simulink model "hitrostni_profili"  (Simulink 8.1)
settings: Solver=ode45  StartTime=0.0  StopTime=1800  MaxStep=1  RelTol=1e-3
values from neighbouring files (symbols this model uses):
  ETC_speed = [0.495937473176 0.496373873447 0.49680642819 0.497232592994 0.497650129408 0.498057004223 0.498451290329 0.498831082365 0.499194437912 0.499539351796 0.499863767467 0.500165625602 ... (17981 elements, 1x17981)]    [ETC_full.mat]
  ETC_time = [1.27562198744 1.37562198744 1.47562198744 1.57562198744 1.67562198744 1.77562198744 1.87562198744 1.97562198744 2.07562198744 2.17562198744 2.27562198744 2.37562198744 ... (17981 elements, 1x17981)]    [ETC_full.mat]
  WMTC_speed = [0.13809804916 0.140640874512 0.143161143435 0.145643612252 0.148074768295 0.150442285099 0.15273449872 0.154939979407 0.157047256677 0.159044735684 0.160920820235 0.162664234602 ... (17997 elements, 1x17997)]    [WMTC_full.mat]
  WMTC_time = [1.06312774212 1.16312774212 1.26312774212 1.36312774212 1.46312774212 1.56312774212 1.66312774212 1.76312774212 1.86312774212 1.96312774212 2.06312774212 2.16312774212 ... (17997 elements, 1x17997)]    [WMTC_full.mat]
libraries: simulink x12
settings Model: Creator=Mitja  LastModifiedBy=MitjaN
settings DebuggingCC: SaveWithParameterizedLinksMsg=none
settings HardwareCC: TargetHWDeviceType=32-bit Generic
settings GRTTargetCC: TargetFcnLib=ansi_tfl_tmw.mat

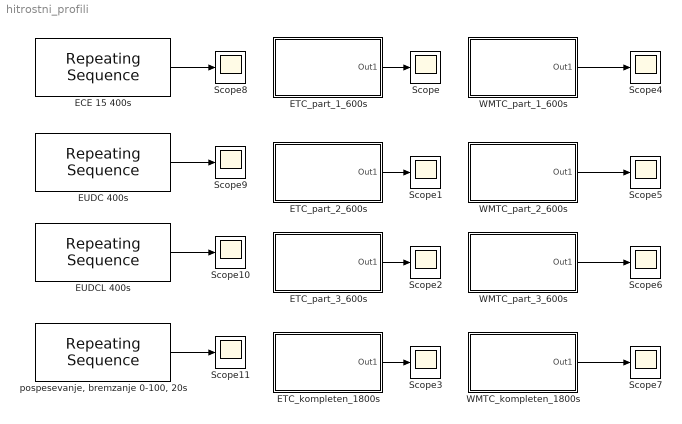
== system hitrostni_profili ==
  ECE 15 400s : simulink/Sources/Repeating Sequence  rep_seq_t=[0.0 11.3 15.0 23.2 28.2 48.9 60.8 85.2 95.9 117.2 142.8 154.8 162.9 176.0 188.0 200.0]  rep_seq_y=[0.0 0.0 5.0 5.0 0.0 0.0 32.0 32.0 0.0 0.0 50.0 50.0 35.0 35.0 0.0 0.0]
  ETC_kompleten_1800s : Subsystem  InitFcn=load('ETC_full.mat')
  ETC_part_1_600s : Subsystem  InitFcn=load('ETC_part_1.mat')
  ETC_part_2_600s : Subsystem  InitFcn=load('ETC_part_2.mat')
  ETC_part_3_600s : Subsystem  InitFcn=load('ETC_part_3.mat')
  EUDC 400s : simulink/Sources/Repeating Sequence  rep_seq_t=[0.0 20.5128 24.359 30.7692 34.6154 43.5897 60.2564 111.538 115.385 119.231 188.462 193.59 194.872 200.0 250.0 284.615 315.385 334.615 346.154 364.103 371.795 379.487 400.0]  rep_seq_y=[0.0 0.0 7.0 19.0 26.0 42.0 70.0 70.0 58.2775 50.0 50.0 58.2775 60.9569 70.0 70.0 100.0 100.0 120.0 120.0 71.0048 37.512 0.0 0.0]
  EUDCL 400s : simulink/Sources/Repeating Sequence  rep_seq_t=|  rep_seq_y=|
      rep_seq_t=|
      | [    0.00000000000000e+000
      |     20.5128000000000e+000
      |     23.0769000000000e+000
      |     28.2051000000000e+000
      |     35.8974000000000e+000
      |     46.1538000000000e+000
      |     61.5385000000000e+000
      |     111.538000000000e+000
      |     115.385000000000e+000
      |     119.231000000000e+000
      |     188.462000000000e+000
      |     193.590000000000e+000
      |     201.282000000000e+000
      |     251.282000000000e+000
      |     274.359000000000e+000
      |     357.692000000000e+000
      |     365.385000000000e+000
      |     379.487000000000e+000
      |     400.000000000000e+000]
      rep_seq_y=|
      | [    0.00000000000000e+000
      |     0.00000000000000e+000
      |     11.0048000000000e+000
      |     18.6603000000000e+000
      |     34.9282000000000e+000
      |     49.7608000000000e+000
      |     70.0000000000000e+000
      |     70.0000000000000e+000
      |     59.3301000000000e+000
      |     50.0000000000000e+000
      |     50.0000000000000e+000
      |     60.2871000000000e+000
      |     70.0000000000000e+000
      |     70.0000000000000e+000
      |     90.0000000000000e+000
      |     90.0000000000000e+000
      |     67.4641000000000e+000
      |     0.00000000000000e+000
      |     0.00000000000000e+000]
  Scope{,1..11} (12 alike) : Scope
      Scope10 settings: SaveName=ScopeData10
      Scope11 settings: SaveName=ScopeData11
      Scope2 settings: SaveName=ScopeData2
      Scope3 settings: SaveName=ScopeData3
      Scope4 settings: SaveName=ScopeData4
      Scope5 settings: SaveName=ScopeData5
      Scope6 settings: SaveName=ScopeData6
      Scope7 settings: SaveName=ScopeData7
      Scope8 settings: SaveName=ScopeData8
      Scope9 settings: SaveName=ScopeData9
  WMTC_kompleten_1800s : Subsystem  InitFcn=load('WMTC_full.mat')
  WMTC_part_1_600s : Subsystem  InitFcn=load('WMTC_part_1.mat')
  WMTC_part_2_600s : Subsystem  InitFcn=load('WMTC_part_2.mat')
  WMTC_part_3_600s : Subsystem  InitFcn=load('WMTC_part_3.mat')
  "pospesevanje, bremzanje 0-100, 20s" : simulink/Sources/Repeating Sequence  rep_seq_t=[0 1 11 15 17 20]  rep_seq_y=[0 0 100 100 0 0]
  wires:
  ETC_part_1_600s/1(Out1) -> Scope/1
  WMTC_kompleten_1800s/1(Out1) -> Scope7/1
  WMTC_part_3_600s/1(Out1) -> Scope6/1
  WMTC_part_2_600s/1(Out1) -> Scope5/1
  WMTC_part_1_600s/1(Out1) -> Scope4/1
  ETC_part_2_600s/1(Out1) -> Scope1/1
  ETC_part_3_600s/1(Out1) -> Scope2/1
  ETC_kompleten_1800s/1(Out1) -> Scope3/1
  ECE 15 400s/1 -> Scope8/1
  EUDC 400s/1 -> Scope9/1
  EUDCL 400s/1 -> Scope10/1
  "pospesevanje, bremzanje 0-100, 20s"/1 -> Scope11/1

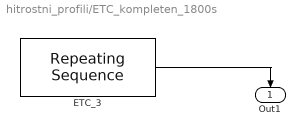
== system hitrostni_profili/ETC_kompleten_1800s ==
  ETC_3 : simulink/Sources/Repeating Sequence  rep_seq_t=[ETC_time]  rep_seq_y=[ETC_speed]
  Out1 : Outport
  wires:
  ETC_3/1 -> Out1/1

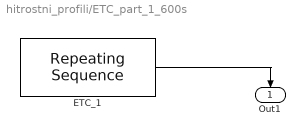
== system hitrostni_profili/ETC_part_1_600s ==
  ETC_1 : simulink/Sources/Repeating Sequence  rep_seq_t=ETC_1_time  rep_seq_y=ETC_1_speed
  Out1 : Outport
  wires:
  ETC_1/1 -> Out1/1

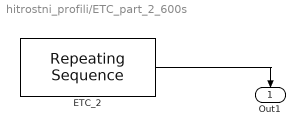
== system hitrostni_profili/ETC_part_2_600s ==
  ETC_2 : simulink/Sources/Repeating Sequence  rep_seq_t=ETC_2_time  rep_seq_y=ETC_2_speed
  Out1 : Outport
  wires:
  ETC_2/1 -> Out1/1

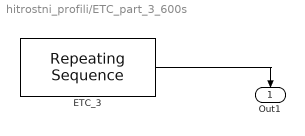
== system hitrostni_profili/ETC_part_3_600s ==
  ETC_3 : simulink/Sources/Repeating Sequence  rep_seq_t=ETC_3_time  rep_seq_y=ETC_3_speed
  Out1 : Outport
  wires:
  ETC_3/1 -> Out1/1

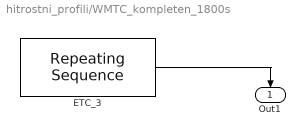
== system hitrostni_profili/WMTC_kompleten_1800s ==
  ETC_3 : simulink/Sources/Repeating Sequence  rep_seq_t=[WMTC_time]  rep_seq_y=[WMTC_speed]
  Out1 : Outport
  wires:
  ETC_3/1 -> Out1/1

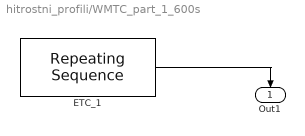
== system hitrostni_profili/WMTC_part_1_600s ==
  ETC_1 : simulink/Sources/Repeating Sequence  rep_seq_t=WMTC_1_time  rep_seq_y=WMTC_1_speed
  Out1 : Outport
  wires:
  ETC_1/1 -> Out1/1

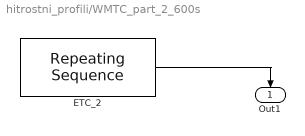
== system hitrostni_profili/WMTC_part_2_600s ==
  ETC_2 : simulink/Sources/Repeating Sequence  rep_seq_t=WMTC_2_time  rep_seq_y=WMTC_2_speed
  Out1 : Outport
  wires:
  ETC_2/1 -> Out1/1

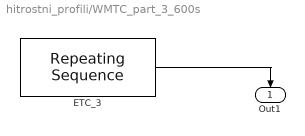
== system hitrostni_profili/WMTC_part_3_600s ==
  ETC_3 : simulink/Sources/Repeating Sequence  rep_seq_t=WMTC_3_time  rep_seq_y=WMTC_3_speed
  Out1 : Outport
  wires:
  ETC_3/1 -> Out1/1
